simulink model "conver"  (R2019b)
settings: Solver=VariableStepAuto  StartTime=0.0  StopTime=10.0  RelTol=1e-3
values from neighbouring files (symbols this model uses):
  C = 10e-6    (= 1e-05)    [run.m]
  e = 10^-2    (= 0.01)    [run.m]
  g = 9.8    [run.m]
  i0 = 13.5    [run.m]
  K_zreal = minreal(-i0/2*(2/(z0+e)+K_z1)*tf([tau_i 1],[1/12500 1]))    [run.m]
  L = 2e-3    (= 0.002)    [run.m]
  m = 100    [run.m]
  R = 10    [run.m]
  z0 = 10^-2    (= 0.01)    [run.m]
  zm = 0.02    [run.m]
undefined symbols (not defined in the file or in its folder): K_i
settings Model: Creator=anasselhoud  LastModifiedBy=anasselhoud

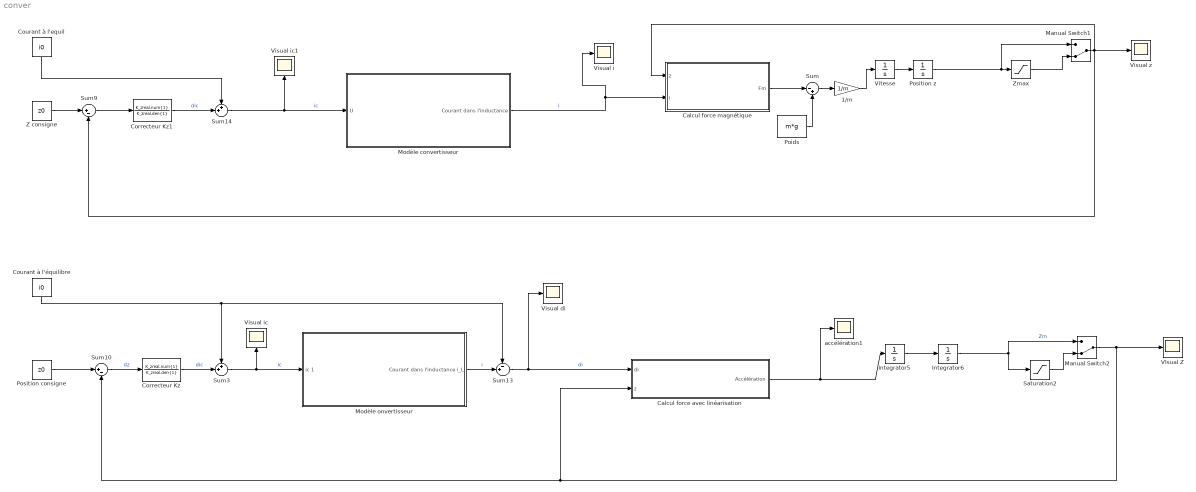
== system conver ==
  1/m : Gain  Gain=1/m
  Calcul force avec linéarisation : Subsystem
  Calcul force magnétique : Subsystem
  Correcteur Kz : TransferFcn  Numerator=K_zreal.num{1}  Denominator=K_zreal.den{1}
  Correcteur Kz1 : TransferFcn  Numerator=K_zreal.num{1}  Denominator=K_zreal.den{1}
  Courant à l'equil : Constant  Value=i0
  Courant à l'équilibre : Constant  Value=i0
  Integrator5 : Integrator
  Integrator6 : Integrator  InitialCondition=2*z0
  Manual Switch1 : ManualSwitch  CurrentSetting=0
  Manual Switch2 : ManualSwitch  CurrentSetting=0
  Modèle convertisseur : Subsystem
  Modèle onvertisseur : Subsystem
  Poids : Constant  Value=m*g
  Position consigne : Constant  Value=z0
  Position z : Integrator  InitialCondition=2*z0
  Saturation2 : Saturate  UpperLimit=zm  LowerLimit=0
  Sum : Sum  Inputs=|-+
  Sum10 : Sum  Inputs=|+-
  Sum13 : Sum  Inputs=-+|
  Sum14 : Sum  Inputs=++|
  Sum3 : Sum  Inputs=++|
  Sum9 : Sum  Inputs=|+-
  VIsual Z : Scope
  Visual di : Scope
  Visual i : Scope
  Visual ic : Scope
  Visual ic1 : Scope
  Visual z : Scope
  Vitesse : Integrator
  Z consigne : Constant  Value=z0
  Zmax : Saturate  UpperLimit=zm  LowerLimit=0
  accélération1 : Scope
  wires:
  Calcul force avec linéarisation/1(Accélération) -> accélération1/1, Integrator5/1
  Correcteur Kz/1 -> Sum3/2  "dic"
  Integrator6/1 -> Saturation2/1, Manual Switch2/1  "Zm"
  Saturation2/1 -> Manual Switch2/2
  Modèle onvertisseur/1(Courant dans l'inductance i_L) -> Sum13/2  "i"
  Manual Switch2/1 -> VIsual Z/1, Calcul force avec linéarisation/2(z), Sum10/2
  Integrator5/1 -> Integrator6/1
  Sum13/1 -> Visual di/1, Calcul force avec linéarisation/1(di)  "di"
  Sum10/1 -> Correcteur Kz/1  "dz"
  Courant à l'équilibre/1 -> Sum13/1, Sum3/1
  Sum3/1 -> Modèle onvertisseur/1(ic 1), Visual ic/1  "ic"
  Position consigne/1 -> Sum10/1
  Calcul force magnétique/1(Fm) -> Sum/1
  Poids/1 -> Sum/2
  1/m/1 -> Vitesse/1
  Sum/1 -> 1/m/1
  Vitesse/1 -> Position z/1
  Position z/1 -> Manual Switch1/1, Zmax/1
  Zmax/1 -> Manual Switch1/2
  Manual Switch1/1 -> Sum9/2, Calcul force magnétique/1(z), Visual z/1
  Courant à l'equil/1 -> Sum14/1
  Sum14/1 -> Visual ic1/1, Modèle convertisseur/1(U)  "ic"
  Correcteur Kz1/1 -> Sum14/2  "dic"
  Sum9/1 -> Correcteur Kz1/1
  Modèle convertisseur/1(Courant dans l'inductance) -> Visual i/1, Calcul force magnétique/2(i)  "i"
  Z consigne/1 -> Sum9/1

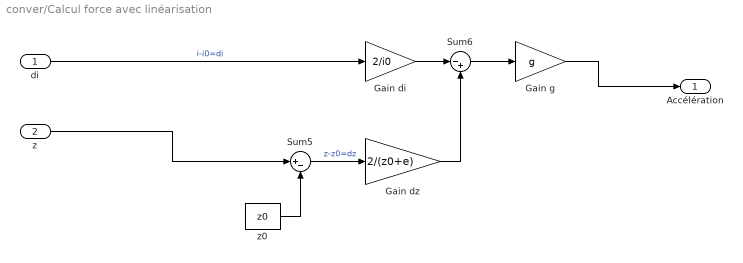
== system conver/Calcul force avec linéarisation ==
  di : Inport
  z : Inport  Port=2
  Gain di : Gain  Gain=2/i0
  Gain dz : Gain  Gain=2/(z0+e)
  Gain g : Gain  Gain=g
  Sum5 : Sum  Inputs=|+-
  Sum6 : Sum  Inputs=|-+
  z0 : Constant  Value=z0
  Accélération : Outport
  wires:
  di/1 -> Gain di/1  "i-i0=di"
  z0/1 -> Sum5/2
  Sum5/1 -> Gain dz/1  "z-z0=dz"
  Gain di/1 -> Sum6/1
  Sum6/1 -> Gain g/1
  Gain dz/1 -> Sum6/2
  Gain g/1 -> Accélération/1
  z/1 -> Sum5/1

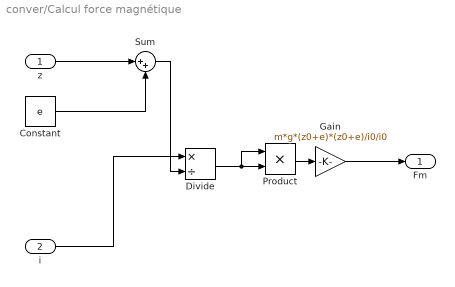
== system conver/Calcul force magnétique ==
  z : Inport
  i : Inport  Port=2
  Constant : Constant  Value=e
  Divide : Product  Inputs=*/
  Gain : Gain  Gain=m*g*(z0+e)*(z0+e)/i0/i0
  Product : Product
  Sum : Sum  Inputs=|++
  Fm : Outport
  wires:
  Product/1 -> Gain/1
  Gain/1 -> Fm/1
  Divide/1 -> Product/1, Product/2
  i/1 -> Divide/1
  Sum/1 -> Divide/2
  z/1 -> Sum/1
  Constant/1 -> Sum/2

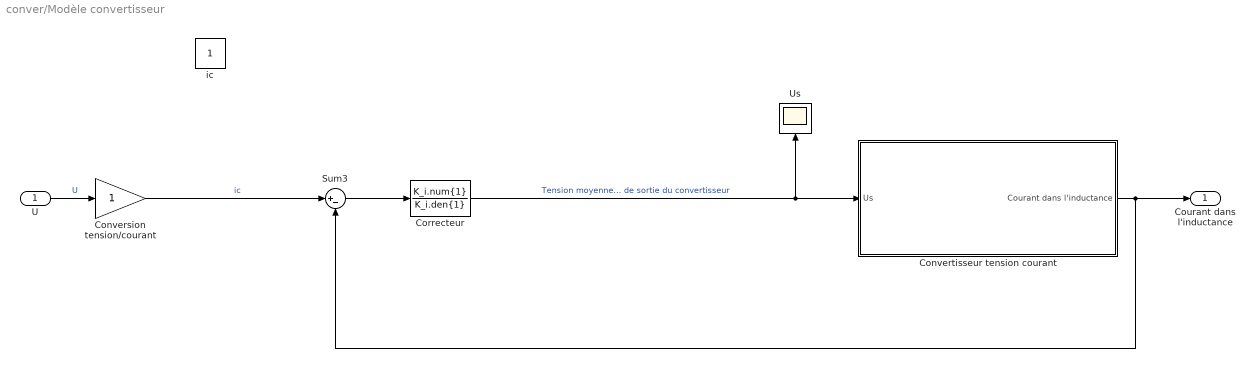
== system conver/Modèle convertisseur ==
  U : Inport
  Conversion tension/courant : Gain
  Convertisseur tension courant : Subsystem
  Correcteur : TransferFcn  Numerator=K_i.num{1}  Denominator=K_i.den{1}
  Sum3 : Sum  Inputs=|+-
  Us : Scope
  ic : Constant
  Courant dans l'inductance : Outport
  wires:
  Correcteur/1 -> Us/1, Convertisseur tension courant/1(Us)  "Tension moyenne de sortie du convertisseur"
  Convertisseur tension courant/1(Courant dans l'inductance) -> Sum3/2, Courant dans l'inductance/1
  U/1 -> Conversion tension/courant/1  "U"
  Conversion tension/courant/1 -> Sum3/1  "ic"
  Sum3/1 -> Correcteur/1

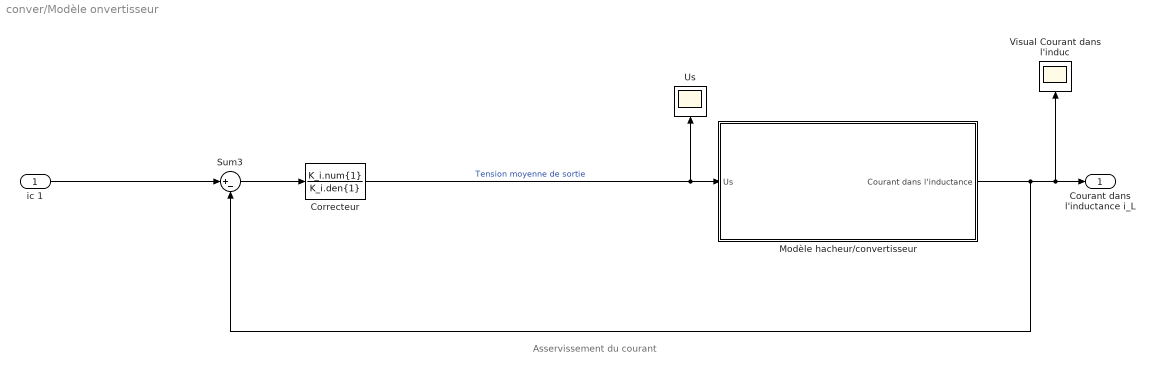
== system conver/Modèle onvertisseur ==
  note: Asservissement du courant
  ic 1 : Inport
  Correcteur : TransferFcn  Numerator=K_i.num{1}  Denominator=K_i.den{1}
  Modèle hacheur/convertisseur : Subsystem
  Sum3 : Sum  Inputs=|+-
  Us : Scope
  Visual Courant dans l'induc : Scope
  Courant dans l'inductance i_L : Outport
  wires:
  Correcteur/1 -> Modèle hacheur/convertisseur/1(Us), Us/1  "Tension moyenne de sortie"
  Modèle hacheur/convertisseur/1(Courant dans l'inductance) -> Visual Courant dans l'induc/1, Courant dans l'inductance i_L/1, Sum3/2
  Sum3/1 -> Correcteur/1
  ic 1/1 -> Sum3/1

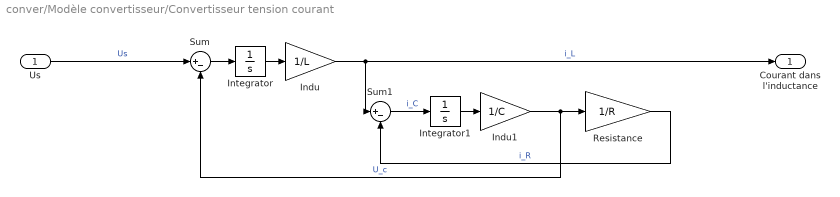
== system conver/Modèle convertisseur/Convertisseur tension courant ==
  Us : Inport
  Indu : Gain  Gain=1/L
  Indu1 : Gain  Gain=1/C
  Integrator : Integrator
  Integrator1 : Integrator
  Resistance : Gain  Gain=1/R
  Sum : Sum  Inputs=|+-
  Sum1 : Sum  Inputs=|+-
  Courant dans l'inductance : Outport
  wires:
  Resistance/1 -> Sum1/2  "i_R"
  Sum1/1 -> Integrator1/1  "i_C"
  Indu1/1 -> Resistance/1, Sum/2  "U_c"
  Indu/1 -> Sum1/1, Courant dans l'inductance/1  "i_L"
  Sum/1 -> Integrator/1
  Integrator/1 -> Indu/1
  Integrator1/1 -> Indu1/1
  Us/1 -> Sum/1  "Us"

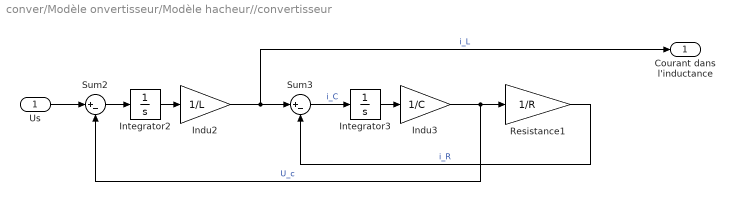
== system conver/Modèle onvertisseur/Modèle hacheur//convertisseur ==
  Us : Inport
  Indu2 : Gain  Gain=1/L
  Indu3 : Gain  Gain=1/C
  Integrator2 : Integrator
  Integrator3 : Integrator
  Resistance1 : Gain  Gain=1/R
  Sum2 : Sum  Inputs=|+-
  Sum3 : Sum  Inputs=|+-
  Courant dans l'inductance : Outport
  wires:
  Integrator3/1 -> Indu3/1
  Indu3/1 -> Resistance1/1, Sum2/2  "U_c"
  Resistance1/1 -> Sum3/2  "i_R"
  Us/1 -> Sum2/1
  Sum2/1 -> Integrator2/1
  Sum3/1 -> Integrator3/1  "i_C"
  Integrator2/1 -> Indu2/1
  Indu2/1 -> Sum3/1, Courant dans l'inductance/1  "i_L"
